simulink model "Skew_correction_1_harness"  (R2020b)
settings: Solver=ode4  StartTime=0.0  StopTime=par.sym.Ttot  FixedStep=0.05  MaxStep=par.sym.max_dt  RelTol=1e-3
settings Model: Creator=carar  LastModifiedBy=carar
settings SolverCC: AlgebraicLoopSolver=LineSearch
settings DataIOCC: SaveOutput=off  SaveTime=off  ReturnWorkspaceOutputs=off  TimeSaveName=TIME
settings OptimizationCC: LifeSpan=inf
settings DebuggingCC: UnconnectedInputMsg=none  UnconnectedOutputMsg=none  ArithmeticOperatorsInVariantConditions=warning
settings SFSimCC: CustomCodeUndefinedFunction=UseInterfaceOnly
settings CodeAppCC: GenerateComments=off
settings SimscapeCC: SimscapeNormalizeSystem=off

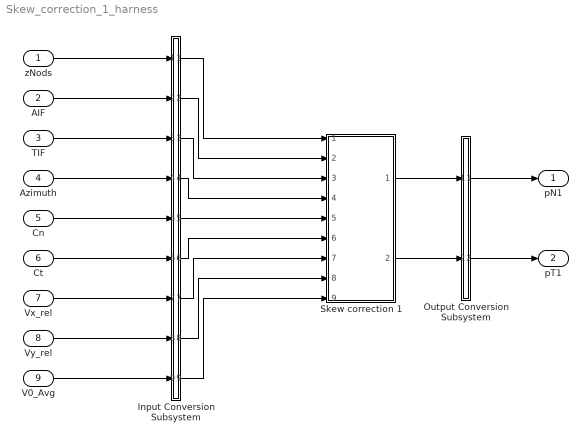
== system Skew_correction_1_harness ==
  zNods : Inport  OutDataTypeStr=double  PortDimensions=[19]  SampleTime=0.05
  AIF : Inport  Port=2  OutDataTypeStr=double  PortDimensions=[19]  SampleTime=0.05
  TIF : Inport  Port=3  OutDataTypeStr=double  PortDimensions=[19]  SampleTime=0.05
  Azimuth : Inport  Port=4  OutDataTypeStr=double  PortDimensions=[1]  SampleTime=0.05
  Cn : Inport  Port=5  OutDataTypeStr=double  PortDimensions=[19]  SampleTime=0.05
  Ct : Inport  Port=6  OutDataTypeStr=double  PortDimensions=[19]  SampleTime=0.05
  Vx_rel : Inport  Port=7  OutDataTypeStr=double  PortDimensions=[19]  SampleTime=0.05
  Vy_rel : Inport  Port=8  OutDataTypeStr=double  PortDimensions=[19]  SampleTime=0.05
  V0_Avg : Inport  Port=9  OutDataTypeStr=double  PortDimensions=[3]  SampleTime=0.05
  Input Conversion Subsystem : Subsystem  Tag=__SLT_ICS__  Description=|
      | Signal spec.
      | and routing
      settings: AttributesFormatString=%<Description>
  Output Conversion Subsystem : Subsystem  Tag=__SLT_OCS__  Description=|
      | Signal spec.
      | and routing
      settings: AttributesFormatString=%<Description>
  Skew correction 1 : ModelReference  ModelNameDialog=Skew_correction_1.slxp  ModelReferenceVersion=5.18  CopyOfModelProtected=on
  pN1 : Outport
  pT1 : Outport  Port=2
  wires:
  zNods/1 -> Input Conversion Subsystem/1(Inport_1)
  AIF/1 -> Input Conversion Subsystem/2(Inport_2)
  TIF/1 -> Input Conversion Subsystem/3(Inport_3)
  Azimuth/1 -> Input Conversion Subsystem/4(Inport_4)
  Cn/1 -> Input Conversion Subsystem/5(Inport_5)
  Ct/1 -> Input Conversion Subsystem/6(Inport_6)
  Vx_rel/1 -> Input Conversion Subsystem/7(Inport_7)
  Vy_rel/1 -> Input Conversion Subsystem/8(Inport_8)
  V0_Avg/1 -> Input Conversion Subsystem/9(Inport_9)
  Output Conversion Subsystem/1(Outport_1) -> pN1/1
  Output Conversion Subsystem/2(Outport_2) -> pT1/1
  Input Conversion Subsystem/1(Outport_1) -> Skew correction 1/1
  Input Conversion Subsystem/2(Outport_2) -> Skew correction 1/2
  Input Conversion Subsystem/3(Outport_3) -> Skew correction 1/3
  Input Conversion Subsystem/4(Outport_4) -> Skew correction 1/4
  Input Conversion Subsystem/5(Outport_5) -> Skew correction 1/5
  Input Conversion Subsystem/6(Outport_6) -> Skew correction 1/6
  Input Conversion Subsystem/7(Outport_7) -> Skew correction 1/7
  Input Conversion Subsystem/8(Outport_8) -> Skew correction 1/8
  Input Conversion Subsystem/9(Outport_9) -> Skew correction 1/9
  Skew correction 1/1 -> Output Conversion Subsystem/1(Inport_1)
  Skew correction 1/2 -> Output Conversion Subsystem/2(Inport_2)

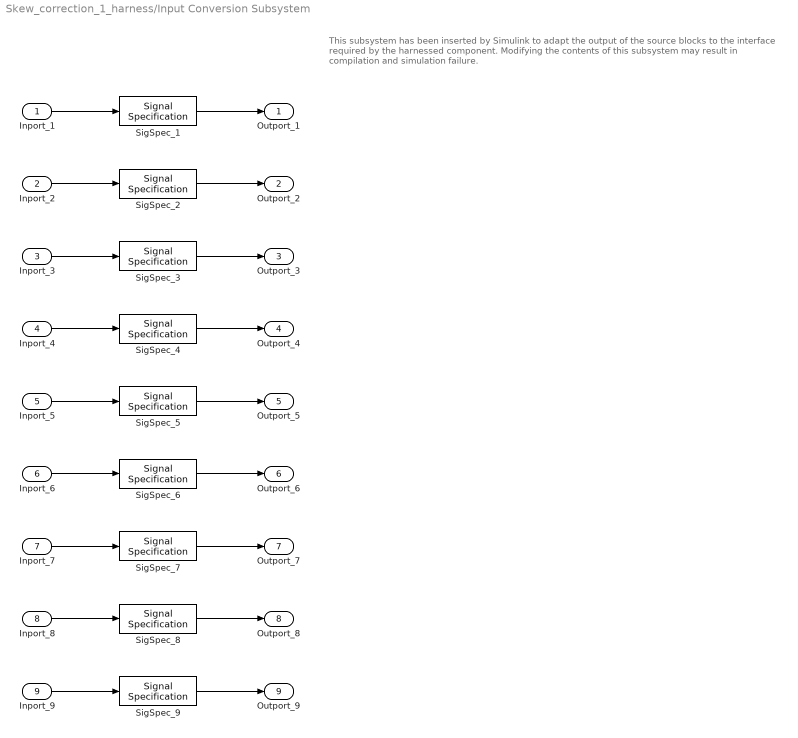
== system Skew_correction_1_harness/Input Conversion Subsystem ==
  note: This subsystem has been inserted by Simulink to adapt the output of the source blocks to the interface required by the harnessed component.
      |  Modifying the contents of this subsystem may result in compilation and simulation failure.
  Inport_1 : Inport
  Inport_2 : Inport  Port=2
  Inport_3 : Inport  Port=3
  Inport_4 : Inport  Port=4
  Inport_5 : Inport  Port=5
  Inport_6 : Inport  Port=6
  Inport_7 : Inport  Port=7
  Inport_8 : Inport  Port=8
  Inport_9 : Inport  Port=9
  SigSpec_{1..3,5..8} (7 alike) : SignalSpecification  OutDataTypeStr=double  Dimensions=[19]  SampleTime=0.05
  SigSpec_4 : SignalSpecification  OutDataTypeStr=double  Dimensions=[1]  SampleTime=0.05
  SigSpec_9 : SignalSpecification  OutDataTypeStr=double  Dimensions=[3]  SampleTime=0.05
  Outport_1 : Outport
  Outport_2 : Outport  Port=2
  Outport_3 : Outport  Port=3
  Outport_4 : Outport  Port=4
  Outport_5 : Outport  Port=5
  Outport_6 : Outport  Port=6
  Outport_7 : Outport  Port=7
  Outport_8 : Outport  Port=8
  Outport_9 : Outport  Port=9
  wires:
  SigSpec_1/1 -> Outport_1/1
  Inport_1/1 -> SigSpec_1/1
  SigSpec_2/1 -> Outport_2/1
  Inport_2/1 -> SigSpec_2/1
  SigSpec_3/1 -> Outport_3/1
  Inport_3/1 -> SigSpec_3/1
  SigSpec_4/1 -> Outport_4/1
  Inport_4/1 -> SigSpec_4/1
  SigSpec_5/1 -> Outport_5/1
  Inport_5/1 -> SigSpec_5/1
  SigSpec_6/1 -> Outport_6/1
  Inport_6/1 -> SigSpec_6/1
  SigSpec_7/1 -> Outport_7/1
  Inport_7/1 -> SigSpec_7/1
  SigSpec_8/1 -> Outport_8/1
  Inport_8/1 -> SigSpec_8/1
  SigSpec_9/1 -> Outport_9/1
  Inport_9/1 -> SigSpec_9/1

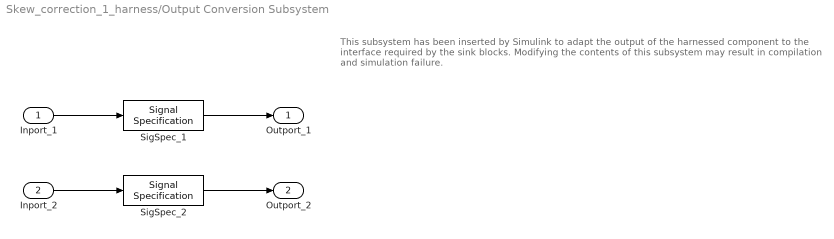
== system Skew_correction_1_harness/Output Conversion Subsystem ==
  note: This subsystem has been inserted by Simulink to adapt the output of the harnessed component to the interface required by the sink blocks.
      |  Modifying the contents of this subsystem may result in compilation and simulation failure.
  Inport_1 : Inport
  Inport_2 : Inport  Port=2
  SigSpec_1 : SignalSpecification  OutDataTypeStr=double  Dimensions=[19]  SampleTime=0.05
  SigSpec_2 : SignalSpecification  OutDataTypeStr=double  Dimensions=[19]  SampleTime=0.05
  Outport_1 : Outport
  Outport_2 : Outport  Port=2
  wires:
  Inport_1/1 -> SigSpec_1/1
  SigSpec_1/1 -> Outport_1/1
  Inport_2/1 -> SigSpec_2/1
  SigSpec_2/1 -> Outport_2/1
